simulink model "untitled1"  (R2019a)
settings: Solver=VariableStepAuto  StartTime=0.0  StopTime=10.0  RelTol=1e-3
libraries: dspsrcs4 x4, dspfdesign x1
settings Model: Creator=timingyang  LastModifiedBy=timingyang

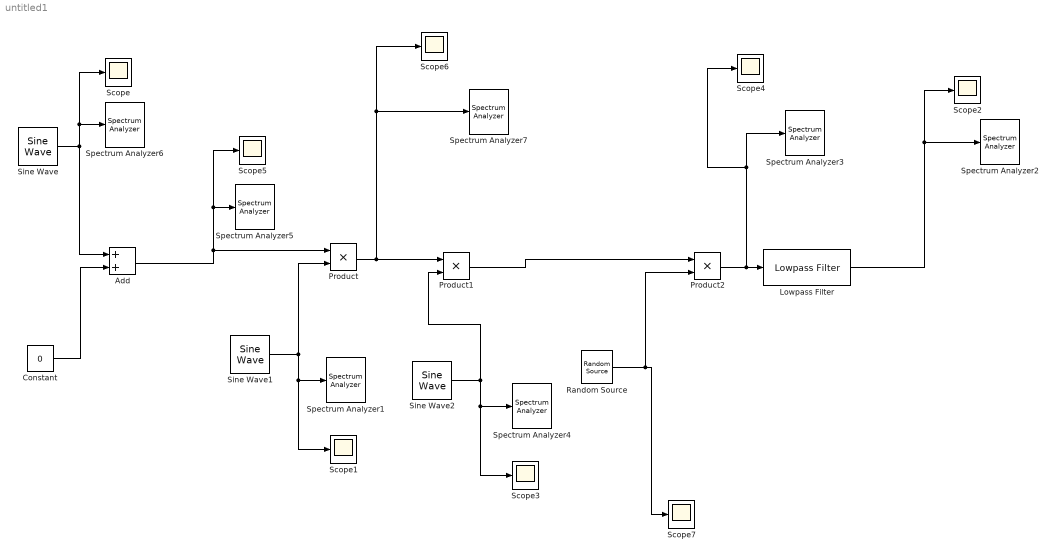
== system untitled1 ==
  Add : Sum
  Constant : Constant  Value=0
  Lowpass Filter : dspfdesign/Lowpass Filter  FilterType=FIR  DesignForMinimumOrder=on  FilterOrder=50  PassbandFrequency=220  StopbandFrequency=300  PassbandRipple=1  StopbandAttenuation=100  InheritSampleRate=off  SampleRate=2000  SimulateUsing=Interpreted execution  roundingMode=Floor  coeffsDataTypeStr=fixdt(1,16)
  Product : Product
  Product1 : Product
  Product2 : Product
  Random Source : dspsrcs4/Random Source  SrcType=Gaussian  NormMethod=Ziggurat  CltLength=12  MinVal=0  MaxVal=1  MeanVal=0  VarVal=1  RepMode=Not repeatable  rawSeed=1  IsInherit=off  SampMode=Discrete  SampTime=1  SampFrame=1  DataType=Double  OutComplex=Real  OutputFrames=off
  Scope{,1..7} (8 alike) : Scope
  Sine Wave : dspsrcs4/Sine Wave  Amplitude=1  Frequency=100  Phase=0  SampleMode=Discrete  OutComplex=Real  CompMethod=Trigonometric fcn  TableSize=Speed  SampleTime=1/2000  SamplesPerFrame=1  ResetState=Restart at time zero  OutputFrames=off  dataType=double  wordLen=16  udDataType=sfix(16)  fracBitsMode=Best precision  numFracBits=15  OutDataTypeStr=double  LastOutDataTypeStr=double
  Sine Wave1 : dspsrcs4/Sine Wave  Amplitude=1  Frequency=300  Phase=0  SampleMode=Discrete  OutComplex=Real  CompMethod=Trigonometric fcn  TableSize=Speed  SampleTime=1/2000  SamplesPerFrame=1  ResetState=Restart at time zero  OutputFrames=off  dataType=double  wordLen=16  udDataType=sfix(16)  fracBitsMode=Best precision  numFracBits=15  OutDataTypeStr=double  LastOutDataTypeStr=double
  Sine Wave2 : dspsrcs4/Sine Wave  Amplitude=1  Frequency=300  Phase=0  SampleMode=Discrete  OutComplex=Real  CompMethod=Trigonometric fcn  TableSize=Speed  SampleTime=1/2000  SamplesPerFrame=1  ResetState=Restart at time zero  OutputFrames=off  dataType=double  wordLen=16  udDataType=sfix(16)  fracBitsMode=Best precision  numFracBits=15  OutDataTypeStr=double  LastOutDataTypeStr=double
  Spectrum Analyzer{1..7} (7 alike) : SpectrumAnalyzer
  wires:
  Sine Wave/1 -> Add/1, Spectrum Analyzer6/1, Scope/1
  Sine Wave1/1 -> Product/2, Spectrum Analyzer1/1, Scope1/1
  Lowpass Filter/1 -> Spectrum Analyzer2/1, Scope2/1
  Constant/1 -> Add/2
  Sine Wave2/1 -> Product1/2, Spectrum Analyzer4/1, Scope3/1
  Add/1 -> Spectrum Analyzer5/1, Scope5/1, Product/1
  Product/1 -> Product1/1, Spectrum Analyzer7/1, Scope6/1
  Product2/1 -> Spectrum Analyzer3/1, Scope4/1, Lowpass Filter/1
  Product1/1 -> Product2/1
  Random Source/1 -> Product2/2, Scope7/1
